simulink model "Modified"  (R2014b)
settings: Solver=ode23s  StartTime=0.0  StopTime=30  FixedStep=0.001  MaxStep=0.01  RelTol=1e-3
StopFcn:
  | plotting
values from neighbouring files (symbols this model uses):
  Par =     [init_params.mat]
undefined symbols (not defined in the file or in its folder): sigbuilder_block
libraries: simulink x4
(part 1 of 2)
settings Model: DSRTSU_INTERNAL_RTI_VER=440  DSRTSU_INTERNAL_RTI_TYPE=rti1401  RTICANMMDATA=struct('GeneralSetupData',struct('modelroot','D:\Users\bengtja\Subversion_work\TM_VEAS_VD\CourseMaterial\MMF062_VehicleDynamics\Compendium\AllPurposeModel','generalsettings',struct('filesettings',struct('destfolder',struct('Name','RTICANMM_FILES','Check',1),'buildfolder',struct('Name','.','Check',1),'AbsDestfolder',struct('Name','D:\Users\bengtja\Subversion_work\TM_VEAS_VD\CourseMaterial\MMF062_VehicleDynamics\Compendium\AllPurposeModel\RTICANMM_FILES'),'AbsBuildfolder',struct('Name','D:\Users\bengtja\Subversion_work\TM_VEAS_VD\CourseMaterial\MMF062_VehicleDynamics\Compendium\AllPurposeModel'))),'options',struct('addpaths',1,'rmpaths',1,'addtrcexclusion',logical(1),'cannavigator',struct('checkmonitoring',0),'show_usrtrc',0,'use_usrtrc',0),'advanced',struct('options',[1 1 1 1 1 1 1 1 1 1 1 1 1 1 1 1 1 1 1 1 1 1 1 1 1 1 1 1 1 1 1 1 1 1 1 1 1 1 1 1 1 1 1 1 1 1 1 1 1 1 1 1 1 1 1 1 1 1 1 1 1 1 1 1 1 1 1 1 1 1 1 1 1 1 1 1 1 1 1 1 1 1 1 1 1 1 1 1 1 1 1 1 1 1 1 1 1 1 1 1]),'MPSetup',{{}},'modelname','AllPurposeModel','block','AllPurposeModel'))  DSRTSU_INTERNAL_RTIFPGA=30  BufferReuse=off  Creator=bengtja  LastModifiedBy=danielpihlquist
settings OptimizationCC: BlockReduction=off  OptimizeBlockIOStorage=off  BufferReuse=off  GlobalBufferReuse=off  ExpressionFolding=off  LocalBlockOutputs=off
settings DebuggingCC: ArtificialAlgebraicLoopMsg=none  UnderspecifiedInitializationDetection=Classic  MergeDetectMultiDrivingBlocksExec=none  StateNameClashWarn=warning
settings HardwareCC: ProdIntDivRoundTo=Zero  ProdEndianess=BigEndian  ProdHWDeviceType=Generic->Custom  TargetIntDivRoundTo=Zero  TargetEndianess=BigEndian  TargetHWDeviceType=Generic->Custom
settings RTWCC: SystemTargetFile=rti1401.tlc  MakeCommand=make_rti  TemplateMakefile=rti1401.tmf  Description=dSPACE DS1401 Hardware Platform  ProcessScript=rti1401_make_rtw_hook
settings STFCustomTargetCC: ParMdlRefBuildCompliant=on  GeneratePreprocessorConditionals=Disable all  MatFileLogging=on  CPPClassGenCompliant=on  SystemTargetFile=rti1401.tlc
settings GRTTargetCC: CompOptLevelCompliant=off  ConcurrentExecutionCompliant=off  CombineOutputUpdateFcns=off  GRTInterface=on  ExtModeMexFile=noextcomm

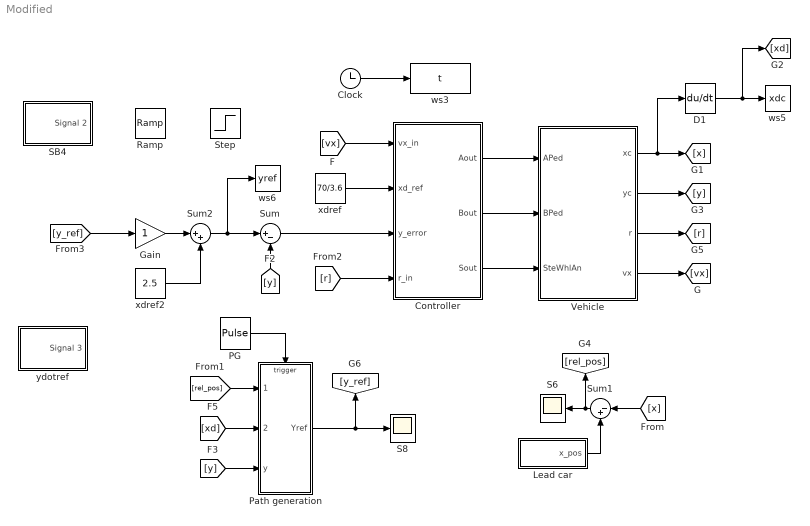
== system Modified ==
  Clock : Clock
  Controller : Subsystem
  D1 : Derivative
  Gain : Gain
  Lead car : Subsystem
  PG : DiscretePulseGenerator  PulseType=Time based  Period=1  PulseWidth=5
  Path generation : Subsystem
  Ramp : simulink/Sources/Ramp  slope=1  start=1  X0=0
  S6 : Scope
      settings: YMin=0  YMax=9  SaveName=ScopeData8
  S8 : Scope
      settings: YMin=0  YMax=9  SaveName=ScopeData10
  SB4 : Subsystem  Tag=STV Subsys  LoadFcn=sigbuilder_block('load');  StartFcn=sigbuilder_block('start');  StopFcn=sigbuilder_block('stop');  ClipboardFcn=sigbuilder_block('clipboard');  mask(Sigbuilder block){}
      mask help: Simulink:masks:SigbuilderBlock_MD
      mask init:
      | if ~strcmp(get_param(bdroot(gcbh),'SimulationStatus'),'stopped') tuvar = sigbuilder_block('maskInit'); end
      settings: CopyFcn=sigbuilder_block('copy');  DeleteFcn=sigbuilder_block('delete');  ModelCloseFcn=sigbuilder_block('modelClose');  PreSaveFcn=sigbuilder_block('preSave');  PauseFcn=sigbuilder_block('pause');  ContinueFcn=sigbuilder_block('continue');  NameChangeFcn=sigbuilder_block('namechange');  OpenFcn=sigbuilder_block('open',[437.6 199.2 550.4 400 ]);  CloseFcn=sigbuilder_block('close');
      mask Display: plot(0, 0, 100, 100,[2, 2, 32, 32, 2], [68, 8, 8, 68, 68],[32, 2], [38, 38], [32, 19, 2],[53, 60, 44], [32, 17, 17, 2],[16, 16, 31, 31]);txt = getActiveGroup(gcbh);text(2, 100, txt,'verticalAlignment', 'top');
  Step : Step  SampleTime=0
  Sum : Sum  Inputs=|+-
  Sum1 : Sum  Inputs=|-+
  Sum2 : Sum  Inputs=|++
  Vehicle : Subsystem
  ws3 : ToWorkspace  VariableName=t  SampleTime=-1
  ws5 : ToWorkspace  VariableName=xdc  SampleTime=-1
  ws6 : ToWorkspace  VariableName=yref  SampleTime=-1
  xdref : Constant  Value=70/3.6
  xdref2 : Constant  Value=2.5
  ydotref : Subsystem  Tag=STV Subsys  LoadFcn=sigbuilder_block('load');  StartFcn=sigbuilder_block('start');  StopFcn=sigbuilder_block('stop');  ClipboardFcn=sigbuilder_block('clipboard');  mask(Sigbuilder block){}
      mask help: Simulink:masks:SigbuilderBlock_MD
      mask init:
      | if ~strcmp(get_param(bdroot(gcbh),'SimulationStatus'),'stopped') tuvar = sigbuilder_block('maskInit'); end
      settings: CopyFcn=sigbuilder_block('copy');  DeleteFcn=sigbuilder_block('delete');  ModelCloseFcn=sigbuilder_block('modelClose');  PreSaveFcn=sigbuilder_block('preSave');  PauseFcn=sigbuilder_block('pause');  ContinueFcn=sigbuilder_block('continue');  NameChangeFcn=sigbuilder_block('namechange');  OpenFcn=sigbuilder_block('open',[437.6 199.2 550.4 400 ]);  CloseFcn=sigbuilder_block('close');
      mask Display: plot(0, 0, 100, 100,[2, 2, 32, 32, 2], [68, 8, 8, 68, 68],[32, 2], [38, 38], [32, 19, 2],[53, 60, 44], [32, 17, 17, 2],[16, 16, 31, 31]);txt = getActiveGroup(gcbh);text(2, 100, txt,'verticalAlignment', 'top');
  wires:
  Clock/1 -> ws3/1
  D1/1 -> ws5/1, [xd]
  Path generation/1(Yref) -> S8/1, [y_ref]
  Sum1/1 -> S6/1, [rel_pos]
  PG/1 -> Path generation/Trigger
  Gain/1 -> Sum2/1
  Sum2/1 -> ws6/1, Sum/1
  xdref2/1 -> Sum2/2
  Lead car/1(x_pos) -> Sum1/2
  xdref/1 -> Controller/2(xd_ref)
  Sum/1 -> Controller/3(y_error)
  [vx] -> Controller/1(vx_in)
  [y] -> Sum/2
  [y] -> Path generation/3(y)
  [xd] -> Path generation/2(xDot)
  [rel_pos] -> Path generation/1(RelPos)
  [r] -> Controller/4(r_in)
  [x] -> Sum1/1
  Vehicle/1(xc) -> D1/1, [x]
  Controller/1(Aout) -> Vehicle/1(APed)
  Controller/2(Bout) -> Vehicle/2(BPed)
  Controller/3(Sout) -> Vehicle/3(SteWhlAn)
  Vehicle/2(yc) -> [y]
  Vehicle/3(r) -> [r]
  Vehicle/4(vx) -> [vx]
  [y_ref] -> Gain/1

== system Modified/Controller ==
  vx_in : Inport
  xd_ref : Inport  Port=2
  y_error : Inport  Port=3
  r_in : Inport  Port=4
  Cartesian controller : Subsystem
  PID2 : simulink/Continuous/PID Controller  Controller=PID  TimeDomain=Continuous-time  SampleTime=-1  IntegratorMethod=Forward Euler  FilterMethod=Forward Euler  Form=Parallel  P=2  I=1  D=0.1  N=0  InitialConditionSource=internal  InitialConditionForIntegrator=0  InitialConditionForFilter=0  ExternalReset=none  LimitOutput=off  UpperSaturationLimit=inf  LowerSaturationLimit=-inf  LinearizeAsGain=on  AntiWindupMode=none  Kb=1  TrackingMode=off  Kt=1  PParamMin=[]  PParamMax=[]  IParamMin=[]  IParamMax=[]  DParamMin=[]  DParamMax=[]  NParamMin=[]  NParamMax=[]  KbParamMin=[]  KbParamMax=[]  KtParamMin=[]  KtParamMax=[]  POutMin=[]  POutMax=[]  IOutMin=[]  IOutMax=[]  DOutMin=[]  DOutMax=[]  NOutMin=[]  NOutMax=[]  KbOutMin=[]  KbOutMax=[]  KtOutMin=[]  KtOutMax=[]  IntegratorOutMin=[]  IntegratorOutMax=[]  FilterOutMin=[]  FilterOutMax=[]  SumOutMin=[]  SumOutMax=[]  SumI1OutMin=[]  SumI1OutMax=[]  SumI2OutMin=[]  SumI2OutMax=[]  SumI3OutMin=[]  SumI3OutMax=[]  SumDOutMin=[]  SumDOutMax=[]  SaturationOutMin=[]  SaturationOutMax=[]  IntegratorContinuousStateAttributes=''  IntegratorStateMustResolveToSignalObject=off  IntegratorRTWStateStorageClass=Auto  FilterContinuousStateAttributes=''  FilterStateMustResolveToSignalObject=off  FilterRTWStateStorageClass=Auto  DifferentiatorICPrevScaledInput=0  DifferentiatorOutMin=[]  DifferentiatorOutMax=[]  UseFilter=on
  Velocity and angle controller : Subsystem
  Aout : Outport
  Bout : Outport  Port=2
  Sout : Outport  Port=3
  wires:
  xd_ref/1 -> Cartesian controller/2(xcd_ref)
  Cartesian controller/2(r_ref) -> Velocity and angle controller/3(r_ref)
  Cartesian controller/1(vx_ref) -> Velocity and angle controller/2(vx_ref)
  r_in/1 -> Velocity and angle controller/4(r_in), Cartesian controller/3(r_in)
  Velocity and angle controller/1(Aout) -> Aout/1
  Velocity and angle controller/2(Bout) -> Bout/1
  Velocity and angle controller/3(Sout) -> Sout/1
  vx_in/1 -> Velocity and angle controller/1(vx_in), Cartesian controller/1(vx_in)
  PID2/1 -> Cartesian controller/4(ycd_ref)
  y_error/1 -> PID2/1

== system Modified/Lead car ==
  Integrator : Integrator  InitialCondition=50
  ws8 : ToWorkspace  VariableName=fcar  SampleTime=-1
  xdref1 : Constant  Value=60/3.6
  x_pos : Outport
  wires:
  xdref1/1 -> Integrator/1
  Integrator/1 -> x_pos/1, ws8/1

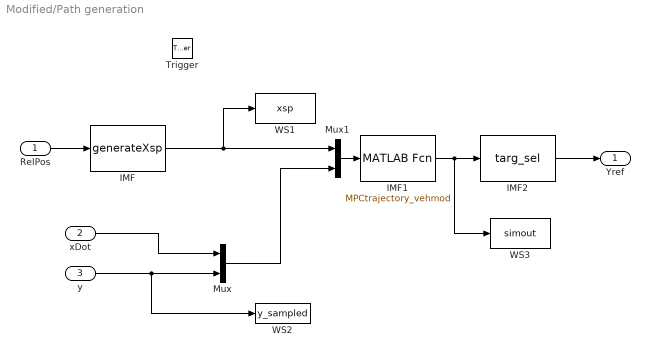
== system Modified/Path generation ==
  RelPos : Inport
  xDot : Inport  Port=2
  y : Inport  Port=3
  Trigger : TriggerPort  PortDimensions=1
  IMF : MATLABFcn  MATLABFcn=generateXsp
  IMF1 : MATLABFcn  MATLABFcn=MPCtrajectory_vehmod
  IMF2 : MATLABFcn  MATLABFcn=targ_sel
  Mux : Mux  Inputs=2
  Mux1 : Mux  Inputs=2
  WS1 : ToWorkspace  VariableName=xsp  SampleTime=-1
  WS2 : ToWorkspace  VariableName=y_sampled  SampleTime=-1
  WS3 : ToWorkspace  VariableName=simout  SampleTime=-1
  Yref : Outport
  wires:
  Mux1/1 -> IMF1/1
  Mux/1 -> Mux1/2
  IMF/1 -> WS1/1, Mux1/1
  RelPos/1 -> IMF/1
  xDot/1 -> Mux/1
  IMF2/1 -> Yref/1
  IMF1/1 -> IMF2/1, WS3/1
  y/1 -> WS2/1, Mux/2

== system Modified/SB4 ==
  Demux : Demux  Tag=STV Demux  Outputs=1
  FromWs : FromWorkspace  Tag=STV FromWs  VariableName=tuvar  SampleTime=0
      SigBuilderData=|
      | common.afterFinalStr = 'Extrapolate'
      | common.sampleTime = 0
      | dataSet.timeRange = [0 10]
      | dataSet.name = 'Group 1'
      | sbobj.Groups.Name = 'Group 1'
      | sbobj.Groups.Signals.Name = 'Signal 2'
      | sbobj.Groups.Signals.XData = [0 0.5 0.5 1 1 1.5 1.5 2 2 2.5 2.5 3 3 3.5 3.5 4 4 4.5 4.5 5 5 5.5 5.5 6 6 6.5 6.5 7 7 7.5 7.5 8 8 8.5 8.5 9 9.5 10]
      | sbobj.Groups.Signals.YData = [0 0 0.275 0.275 0.58 0.58 1 1 1.005 1.005 0.995 0.995 0.745 0.745 0.505 0.505 0.18 0.18 -0.305 -0.305 -0.425 -0.425 -0.56 -0.56 -0.52 -0.52 -0.46 -0.46 -0.43 -0.43 -0.28 -0.28 -0.21 -0.21 0 0 0 0]
  Signal 2 : Outport  Tag=STV Outport
  wires:
  Demux/1 -> Signal 2/1
  FromWs/1 -> Demux/1

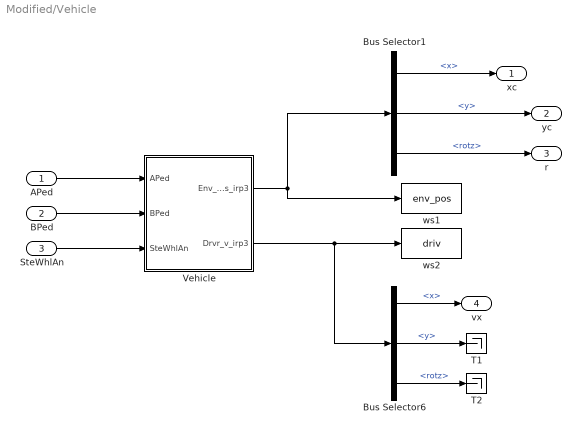
== system Modified/Vehicle ==
  APed : Inport
  BPed : Inport  Port=2
  SteWhlAn : Inport  Port=3
  Bus Selector1 : BusSelector  OutputSignals=x,y,rotz
  Bus Selector6 : BusSelector  OutputSignals=x,y,rotz
  T1 : Terminator
  T2 : Terminator
  Vehicle : Subsystem
  ws1 : ToWorkspace  VariableName=env_pos  SaveFormat=Timeseries  SampleTime=-1
  ws2 : ToWorkspace  VariableName=driv  SaveFormat=Timeseries  SampleTime=-1
  xc : Outport
  yc : Outport  Port=2
  r : Outport  Port=3
  vx : Outport  Port=4
  wires:
  Bus Selector1/1 -> xc/1  "<x>"
  Vehicle/1(Env_pos_irp3) -> Bus Selector1/1, ws1/1
  Vehicle/2(Drvr_v_irp3) -> ws2/1, Bus Selector6/1
  Bus Selector1/2 -> yc/1  "<y>"
  SteWhlAn/1 -> Vehicle/3(SteWhlAn)
  BPed/1 -> Vehicle/2(BPed)
  APed/1 -> Vehicle/1(APed)
  Bus Selector1/3 -> r/1  "<rotz>"
  Bus Selector6/1 -> vx/1  "<x>"
  Bus Selector6/2 -> T1/1  "<y>"
  Bus Selector6/3 -> T2/1  "<rotz>"

== system Modified/ydotref ==
  Demux : Demux  Tag=STV Demux  Outputs=1
  FromWs : FromWorkspace  Tag=STV FromWs  VariableName=tuvar  SampleTime=0
      SigBuilderData=|
      | common.afterFinalStr = 'Extrapolate'
      | common.sampleTime = 0
      | dataSet.timeRange = [0 10]
      | dataSet.name = 'Group 1'
      | sbobj.Groups.Name = 'Group 1'
      | sbobj.Groups.Signals.Name = 'Signal 3'
      | sbobj.Groups.Signals.XData = [0 0.5 0.5 6.8 7.9 8.3 9.26 10]
      | sbobj.Groups.Signals.YData = [0 0 1 1 1 1 1 1]
  Signal 3 : Outport  Tag=STV Outport
  wires:
  Demux/1 -> Signal 3/1
  FromWs/1 -> Demux/1

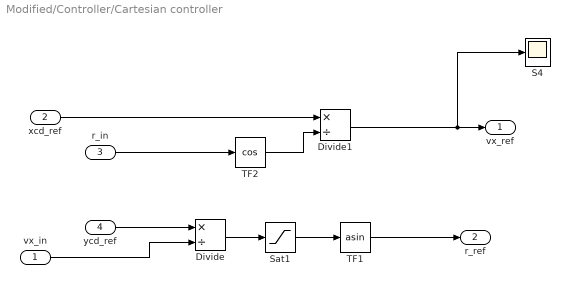
== system Modified/Controller/Cartesian controller ==
  vx_in : Inport
  xcd_ref : Inport  Port=2
  r_in : Inport  Port=3
  ycd_ref : Inport  Port=4
  Divide : Product  Inputs=*/
  Divide1 : Product  Inputs=*/
  S4 : Scope
      settings: SaveName=ScopeData4
  Sat1 : Saturate  UpperLimit=1  LowerLimit=-1
  TF1 : Trigonometry  Operator=asin
  TF2 : Trigonometry  Operator=cos
  vx_ref : Outport
  r_ref : Outport  Port=2
  wires:
  xcd_ref/1 -> Divide1/1
  TF2/1 -> Divide1/2
  r_in/1 -> TF2/1
  vx_in/1 -> Divide/2
  Divide/1 -> Sat1/1
  TF1/1 -> r_ref/1
  Sat1/1 -> TF1/1
  ycd_ref/1 -> Divide/1
  Divide1/1 -> S4/1, vx_ref/1

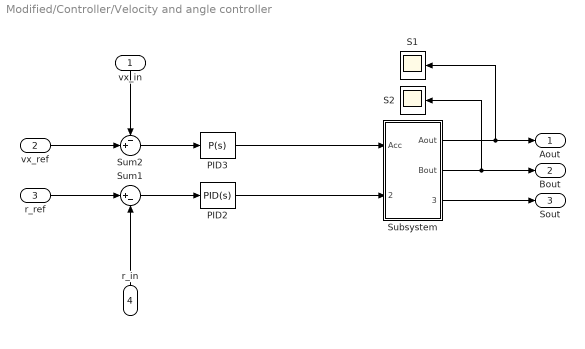
== system Modified/Controller/Velocity and angle controller ==
  vx_in : Inport
  vx_ref : Inport  Port=2
  r_ref : Inport  Port=3
  r_in : Inport  Port=4
  PID2 : simulink/Continuous/PID Controller  Controller=PID  TimeDomain=Continuous-time  SampleTime=-1  IntegratorMethod=Forward Euler  FilterMethod=Forward Euler  Form=Parallel  P=5000  I=1  D=0  N=100  InitialConditionSource=internal  InitialConditionForIntegrator=0  InitialConditionForFilter=0  ExternalReset=none  LimitOutput=off  UpperSaturationLimit=inf  LowerSaturationLimit=-inf  LinearizeAsGain=on  AntiWindupMode=none  Kb=1  TrackingMode=off  Kt=1  PParamMin=[]  PParamMax=[]  IParamMin=[]  IParamMax=[]  DParamMin=[]  DParamMax=[]  NParamMin=[]  NParamMax=[]  KbParamMin=[]  KbParamMax=[]  KtParamMin=[]  KtParamMax=[]  POutMin=[]  POutMax=[]  IOutMin=[]  IOutMax=[]  DOutMin=[]  DOutMax=[]  NOutMin=[]  NOutMax=[]  KbOutMin=[]  KbOutMax=[]  KtOutMin=[]  KtOutMax=[]  IntegratorOutMin=[]  IntegratorOutMax=[]  FilterOutMin=[]  FilterOutMax=[]  SumOutMin=[]  SumOutMax=[]  SumI1OutMin=[]  SumI1OutMax=[]  SumI2OutMin=[]  SumI2OutMax=[]  SumI3OutMin=[]  SumI3OutMax=[]  SumDOutMin=[]  SumDOutMax=[]  SaturationOutMin=[]  SaturationOutMax=[]  IntegratorContinuousStateAttributes=''  IntegratorStateMustResolveToSignalObject=off  IntegratorRTWStateStorageClass=Auto  FilterContinuousStateAttributes=''  FilterStateMustResolveToSignalObject=off  FilterRTWStateStorageClass=Auto  DifferentiatorICPrevScaledInput=0  DifferentiatorOutMin=[]  DifferentiatorOutMax=[]  UseFilter=on
  PID3 : simulink/Continuous/PID Controller  Controller=P  TimeDomain=Continuous-time  SampleTime=-1  IntegratorMethod=Forward Euler  FilterMethod=Forward Euler  Form=Parallel  P=100  I=0  D=0  N=100  InitialConditionSource=internal  InitialConditionForIntegrator=0  InitialConditionForFilter=0  ExternalReset=none  LimitOutput=off  UpperSaturationLimit=inf  LowerSaturationLimit=-inf  LinearizeAsGain=on  AntiWindupMode=none  Kb=1  TrackingMode=off  Kt=1  PParamMin=[]  PParamMax=[]  IParamMin=[]  IParamMax=[]  DParamMin=[]  DParamMax=[]  NParamMin=[]  NParamMax=[]  KbParamMin=[]  KbParamMax=[]  KtParamMin=[]  KtParamMax=[]  POutMin=[]  POutMax=[]  IOutMin=[]  IOutMax=[]  DOutMin=[]  DOutMax=[]  NOutMin=[]  NOutMax=[]  KbOutMin=[]  KbOutMax=[]  KtOutMin=[]  KtOutMax=[]  IntegratorOutMin=[]  IntegratorOutMax=[]  FilterOutMin=[]  FilterOutMax=[]  SumOutMin=[]  SumOutMax=[]  SumI1OutMin=[]  SumI1OutMax=[]  SumI2OutMin=[]  SumI2OutMax=[]  SumI3OutMin=[]  SumI3OutMax=[]  SumDOutMin=[]  SumDOutMax=[]  SaturationOutMin=[]  SaturationOutMax=[]  IntegratorContinuousStateAttributes=''  IntegratorStateMustResolveToSignalObject=off  IntegratorRTWStateStorageClass=Auto  FilterContinuousStateAttributes=''  FilterStateMustResolveToSignalObject=off  FilterRTWStateStorageClass=Auto  DifferentiatorICPrevScaledInput=0  DifferentiatorOutMin=[]  DifferentiatorOutMax=[]  UseFilter=on
  S1 : Scope
      settings: YMin=0  YMax=9  SaveName=ScopeData6
  S2 : Scope
      settings: YMin=0  YMax=9  SaveName=ScopeData7
  Subsystem : Subsystem
  Sum1 : Sum  Inputs=|+-
  Sum2 : Sum  Inputs=-+|
  Aout : Outport
  Bout : Outport  Port=2
  Sout : Outport  Port=3
  wires:
  r_in/1 -> Sum1/2
  Sum1/1 -> PID2/1
  r_ref/1 -> Sum1/1
  Sum2/1 -> PID3/1
  vx_ref/1 -> Sum2/2
  vx_in/1 -> Sum2/1
  Subsystem/2(Bout) -> S2/1, Bout/1
  PID2/1 -> Subsystem/2(Steer)
  Subsystem/3(SOut) -> Sout/1
  PID3/1 -> Subsystem/1(Acc)
  Subsystem/1(Aout) -> S1/1, Aout/1

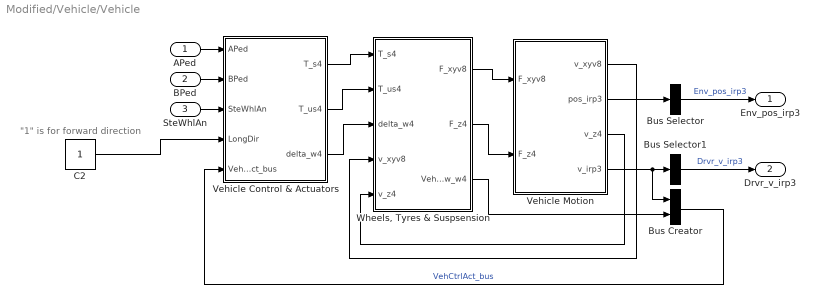
== system Modified/Vehicle/Vehicle ==
  note: "1" is for forward direction
  APed : Inport
  BPed : Inport  Port=2
  SteWhlAn : Inport  Port=3
  Bus Creator : BusCreator  Inputs=2
  Bus Selector : BusSelector  OutputSignals=x,y,rotz  OutputAsBus=on
  Bus Selector1 : BusSelector  OutputSignals=x,y,rotz  OutputAsBus=on
  C2 : Constant
  Vehicle Control & Actuators : Subsystem
  Vehicle Motion : Subsystem
  "Wheels, Tyres & Suspsension" : Subsystem
  Env_pos_irp3 : Outport
  Drvr_v_irp3 : Outport  Port=2
  wires:
  Vehicle Motion/2(pos_irp3) -> Bus Selector/1
  BPed/1 -> Vehicle Control & Actuators/2(BPed)
  SteWhlAn/1 -> Vehicle Control & Actuators/3(SteWhlAn)
  APed/1 -> Vehicle Control & Actuators/1(APed)
  Vehicle Control & Actuators/2(T_us4) -> "Wheels, Tyres & Suspsension"/2(T_us4)
  Vehicle Control & Actuators/1(T_s4) -> "Wheels, Tyres & Suspsension"/1(T_s4)
  Vehicle Control & Actuators/3(delta_w4) -> "Wheels, Tyres & Suspsension"/3(delta_w4)
  "Wheels, Tyres & Suspsension"/1(F_xyv8) -> Vehicle Motion/1(F_xyv8)
  "Wheels, Tyres & Suspsension"/2(F_z4) -> Vehicle Motion/2(F_z4)
  Vehicle Motion/1(v_xyv8) -> "Wheels, Tyres & Suspsension"/4(v_xyv8)
  Vehicle Motion/3(v_z4) -> "Wheels, Tyres & Suspsension"/5(v_z4)
  Vehicle Motion/4(v_irp3) -> Bus Creator/1, Bus Selector1/1
  "Wheels, Tyres & Suspsension"/3(VehCtrlAct_w_w4) -> Bus Creator/2
  Bus Creator/1 -> Vehicle Control & Actuators/5(VehCtrlAct_bus)  "VehCtrlAct_bus"
  Bus Selector/1 -> Env_pos_irp3/1  "Env_pos_irp3"
  Bus Selector1/1 -> Drvr_v_irp3/1  "Drvr_v_irp3"
  C2/1 -> Vehicle Control & Actuators/4(LongDir)

== system Modified/Controller/Velocity and angle controller/Subsystem ==
  Acc : Inport
  Steer : Inport  Port=2
  Gain : Gain  Gain=2/300
  Sat1 : Saturate  UpperLimit=10  LowerLimit=-10
  Sat2 : Saturate  UpperLimit=0  LowerLimit=-1
  Sat3 : Saturate  UpperLimit=1  LowerLimit=0
  Aout : Outport
  Bout : Outport  Port=2
  SOut : Outport  Port=3
  wires:
  Sat1/1 -> SOut/1
  Gain/1 -> Sat1/1
  Steer/1 -> Gain/1
  Acc/1 -> Sat3/1, Sat2/1
  Sat3/1 -> Aout/1
  Sat2/1 -> Bout/1

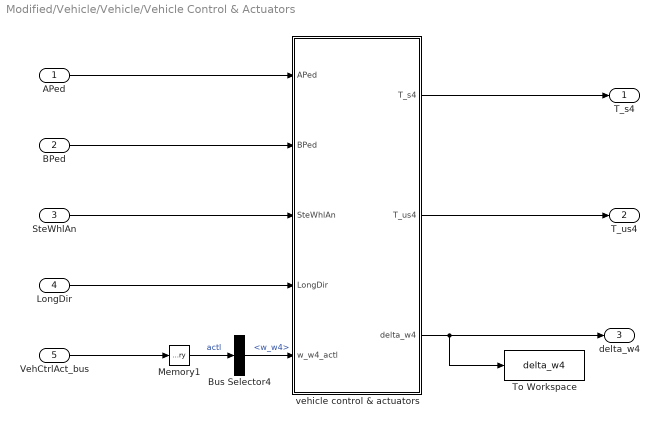
== system Modified/Vehicle/Vehicle/Vehicle Control & Actuators ==
  APed : Inport
  BPed : Inport  Port=2
  SteWhlAn : Inport  Port=3
  LongDir : Inport  Port=4
  VehCtrlAct_bus : Inport  Port=5
  Bus Selector4 : BusSelector  OutputSignals=VehCtrlAct_w_w4.w_w4
  Memory1 : Memory  X0=Par.Init.v_x
  To Workspace : ToWorkspace  VariableName=delta_w4  SaveFormat=Timeseries  SampleTime=-1
  vehicle control & actuators : MATLAB Function  TreatAsAtomicUnit=on
      settings: MinAlgLoopOccurrences=on
  T_s4 : Outport
  T_us4 : Outport  Port=2
  delta_w4 : Outport  Port=3
  wires:
  APed/1 -> vehicle control & actuators/1(APed)
  vehicle control & actuators/2(T_us4) -> T_us4/1
  BPed/1 -> vehicle control & actuators/2(BPed)
  SteWhlAn/1 -> vehicle control & actuators/3(SteWhlAn)
  vehicle control & actuators/1(T_s4) -> T_s4/1
  vehicle control & actuators/3(delta_w4) -> To Workspace/1, delta_w4/1
  VehCtrlAct_bus/1 -> Memory1/1
  Bus Selector4/1 -> vehicle control & actuators/5(w_w4_actl)  "<w_w4>"
  LongDir/1 -> vehicle control & actuators/4(LongDir)
  Memory1/1 -> Bus Selector4/1  "actl"

== system Modified/Vehicle/Vehicle/Vehicle Motion ==
  note: "Sprung Body OORP" could also output pos_oorp3 by integrating v_oorp3.
  F_xyv8 : Inport
  F_z4 : Inport  Port=2
  Compatibility IRP : Subsystem
  Compatibility OORP : Subsystem
  Sprung Body OORP : Subsystem
  Whole Vehicle IRP : Subsystem
  v_xyv8 : Outport
  pos_irp3 : Outport  Port=2
  v_z4 : Outport  Port=3
  v_irp3 : Outport  Port=4
  wires:
  F_xyv8/1 -> Whole Vehicle IRP/1(F_xyv8), Sprung Body OORP/1(F_xyv8)
  F_z4/1 -> Sprung Body OORP/2(F_z4)
  Sprung Body OORP/1(v_oorp3) -> Compatibility OORP/1(v_oorp3)
  Compatibility OORP/1(v_z4) -> v_z4/1
  Compatibility IRP/1(v_xyv8) -> v_xyv8/1
  Whole Vehicle IRP/1(v_irp3) -> v_irp3/1, Compatibility IRP/1(v_irp3)
  Whole Vehicle IRP/2(pos_irp3) -> pos_irp3/1

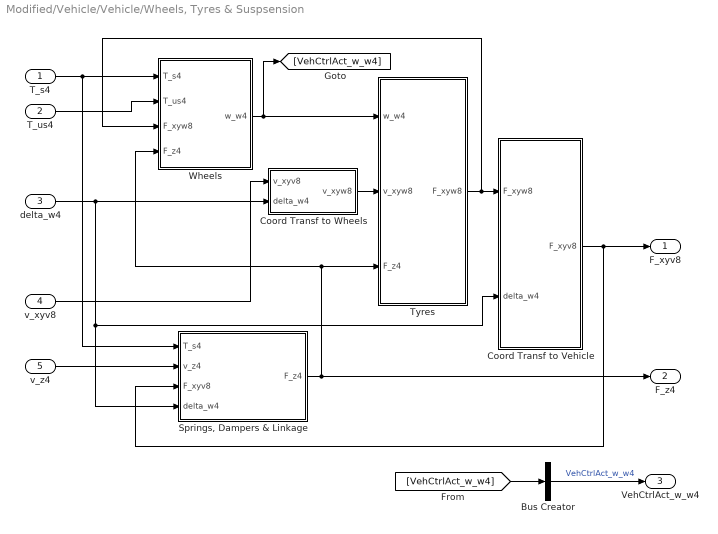
== system Modified/Vehicle/Vehicle/Wheels, Tyres & Suspsension ==
  T_s4 : Inport
  T_us4 : Inport  Port=2
  delta_w4 : Inport  Port=3
  v_xyv8 : Inport  Port=4
  v_z4 : Inport  Port=5
  Bus Creator : BusCreator  Inputs=1
  Coord Transf to Vehicle : Subsystem
      settings: MinAlgLoopOccurrences=on
  "Coord Transf to Wheels " : Subsystem
      settings: MinAlgLoopOccurrences=on
  "Springs, Dampers & Linkage" : Subsystem
      settings: MinAlgLoopOccurrences=on
  "Tyres " : Subsystem
      settings: MinAlgLoopOccurrences=on
  "Wheels " : Subsystem
      settings: MinAlgLoopOccurrences=on
  F_xyv8 : Outport
  F_z4 : Outport  Port=2
  VehCtrlAct_w_w4 : Outport  Port=3
  wires:
  "Tyres "/1(F_xyw8) -> "Wheels "/3(F_xyw8), Coord Transf to Vehicle/1(F_xyw8)
  "Coord Transf to Wheels "/1(v_xyw8) -> "Tyres "/2(v_xyw8)
  delta_w4/1 -> "Springs, Dampers & Linkage"/4(delta_w4), Coord Transf to Vehicle/2(delta_w4), "Coord Transf to Wheels "/2(delta_w4)
  "Wheels "/1(w_w4) -> [VehCtrlAct_w_w4], "Tyres "/1(w_w4)
  T_us4/1 -> "Wheels "/2(T_us4)
  v_xyv8/1 -> "Coord Transf to Wheels "/1(v_xyv8)
  Bus Creator/1 -> VehCtrlAct_w_w4/1  "VehCtrlAct_w_w4"
  [VehCtrlAct_w_w4] -> Bus Creator/1
  v_z4/1 -> "Springs, Dampers & Linkage"/2(v_z4)
  T_s4/1 -> "Springs, Dampers & Linkage"/1(T_s4), "Wheels "/1(T_s4)
  Coord Transf to Vehicle/1(F_xyv8) -> F_xyv8/1, "Springs, Dampers & Linkage"/3(F_xyv8)
  "Springs, Dampers & Linkage"/1(F_z4) -> F_z4/1, "Tyres "/3(F_z4), "Wheels "/4(F_z4)

== system Modified/Vehicle/Vehicle/Vehicle Motion/Compatibility IRP ==
  v_irp3 : Inport
  Bus Creator3 : BusCreator  Inputs=2
  Compatibility : MATLAB Function  TreatAsAtomicUnit=on
  To Workspace1 : ToWorkspace  VariableName=v_xv4  SaveFormat=Timeseries  SampleTime=-1
  To Workspace2 : ToWorkspace  VariableName=v_yv4  SaveFormat=Timeseries  SampleTime=-1
  v_xyv8 : Outport
  wires:
  v_irp3/1 -> Compatibility/1(v_irp3)
  Compatibility/1(v_xv4) -> Bus Creator3/1, To Workspace1/1
  Compatibility/2(v_yv4) -> Bus Creator3/2, To Workspace2/1
  Bus Creator3/1 -> v_xyv8/1  "v_xyv8"

== system Modified/Vehicle/Vehicle/Vehicle Motion/Compatibility OORP ==
  v_oorp3 : Inport
  Compatibility Eq [1.11] : MATLAB Function  TreatAsAtomicUnit=on
  v_z4 : Outport
  wires:
  v_oorp3/1 -> Compatibility Eq [1.11]/1(v_oorp3)
  Compatibility Eq [1.11]/1(v_z4) -> v_z4/1

== system Modified/Vehicle/Vehicle/Vehicle Motion/Sprung Body OORP ==
  F_xyv8 : Inport
  F_z4 : Inport  Port=2
  Body OORP : MATLAB Function  TreatAsAtomicUnit=on
  Bus Selector1 : BusSelector  OutputSignals=F_xv4,F_yv4
  Integrator : Subsystem
  v_oorp3 : Outport
  wires:
  F_z4/1 -> Body OORP/3(F_z4)
  Body OORP/1(derv_oorp3) -> Integrator/1(derv_z)
  Integrator/1(v_oorp3) -> v_oorp3/1
  F_xyv8/1 -> Bus Selector1/1
  Bus Selector1/1 -> Body OORP/1(F_xv4)  "<F_xv4>"
  Bus Selector1/2 -> Body OORP/2(F_yv4)  "<F_yv4>"

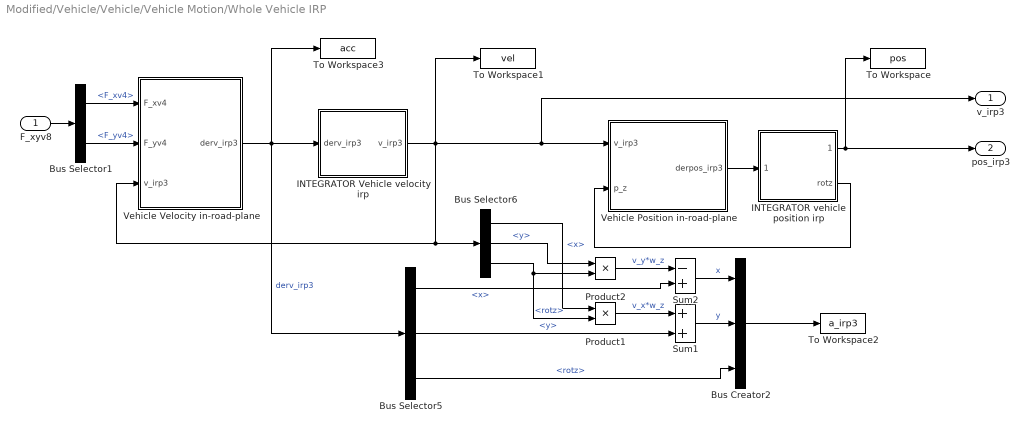
== system Modified/Vehicle/Vehicle/Vehicle Motion/Whole Vehicle IRP ==
  F_xyv8 : Inport
  Bus Creator2 : BusCreator  Inputs=3  OutDataTypeStr=Bus: irp_vec3
  Bus Selector1 : BusSelector  OutputSignals=F_xv4,F_yv4
  Bus Selector5 : BusSelector  OutputSignals=x,y,rotz
  Bus Selector6 : BusSelector  OutputSignals=x,y,rotz
  INTEGRATOR Vehicle velocity irp : Subsystem
  INTEGRATOR vehicle position irp : Subsystem
  Product1 : Product
  Product2 : Product
  Sum1 : Sum
  Sum2 : Sum  Inputs=-+
  To Workspace : ToWorkspace  VariableName=pos  SaveFormat=Timeseries  SampleTime=-1
  To Workspace1 : ToWorkspace  VariableName=vel  SaveFormat=Timeseries  SampleTime=-1
  To Workspace2 : ToWorkspace  VariableName=a_irp3  SaveFormat=Timeseries  SampleTime=-1
  To Workspace3 : ToWorkspace  VariableName=acc  SaveFormat=Timeseries  SampleTime=-1
  Vehicle Position in-road-plane : MATLAB Function  TreatAsAtomicUnit=on
  Vehicle Velocity in-road-plane : MATLAB Function  TreatAsAtomicUnit=on
  v_irp3 : Outport
  pos_irp3 : Outport  Port=2
  wires:
  Bus Creator2/1 -> To Workspace2/1
  Product1/1 -> Sum1/1  "v_x*w_z"
  Sum1/1 -> Bus Creator2/2  "y"
  Sum2/1 -> Bus Creator2/1  "x"
  Product2/1 -> Sum2/1  "v_y*w_z"
  Vehicle Velocity in-road-plane/1(derv_irp3) -> To Workspace3/1, Bus Selector5/1, INTEGRATOR Vehicle velocity irp/1(derv_irp3)  "derv_irp3"
  INTEGRATOR Vehicle velocity irp/1(v_irp3) -> Vehicle Position in-road-plane/1(v_irp3), v_irp3/1, Bus Selector6/1, Vehicle Velocity in-road-plane/3(v_irp3), To Workspace1/1
  Bus Selector5/3 -> Bus Creator2/3  "<rotz>"
  Bus Selector5/2 -> Sum1/2  "<y>"
  Bus Selector5/1 -> Sum2/2  "<x>"
  Bus Selector6/2 -> Product2/1  "<y>"
  Bus Selector6/3 -> Product2/2, Product1/2  "<rotz>"
  Bus Selector6/1 -> Product1/1  "<x>"
  INTEGRATOR vehicle position irp/1(pos_irp3) -> To Workspace/1, pos_irp3/1
  Vehicle Position in-road-plane/1(derpos_irp3) -> INTEGRATOR vehicle position irp/1(derpos_irp3)
  INTEGRATOR vehicle position irp/2(rotz) -> Vehicle Position in-road-plane/2(p_z)
  F_xyv8/1 -> Bus Selector1/1
  Bus Selector1/1 -> Vehicle Velocity in-road-plane/1(F_xv4)  "<F_xv4>"
  Bus Selector1/2 -> Vehicle Velocity in-road-plane/2(F_yv4)  "<F_yv4>"

== system Modified/Vehicle/Vehicle/Wheels, Tyres & Suspsension/Coord Transf to Vehicle ==
  F_xyw8 : Inport
  delta_w4 : Inport  Port=2
  Bus Creator3 : BusCreator  Inputs=2
  Bus Selector1 : BusSelector  OutputSignals=F_xw4,F_yw4
  Coord Transf to veh : MATLAB Function  TreatAsAtomicUnit=on
      settings: MinAlgLoopOccurrences=on
  F_xyv8 : Outport
  wires:
  delta_w4/1 -> Coord Transf to veh/3(delta_w4)
  Coord Transf to veh/1(F_xv4) -> Bus Creator3/1
  Coord Transf to veh/2(F_yv4) -> Bus Creator3/2
  F_xyw8/1 -> Bus Selector1/1
  Bus Creator3/1 -> F_xyv8/1  "F_xyv8"
  Bus Selector1/1 -> Coord Transf to veh/1(F_xw4)  "<F_xw4>"
  Bus Selector1/2 -> Coord Transf to veh/2(F_yw4)  "<F_yw4>"

== system Modified/Vehicle/Vehicle/Wheels, Tyres & Suspsension/Coord Transf to Wheels  ==
  v_xyv8 : Inport
  delta_w4 : Inport  Port=2
  Bus Creator4 : BusCreator  Inputs=2
  Bus Selector : BusSelector  OutputSignals=v_xv4,v_yv4
  Coord Transf to whl : MATLAB Function  TreatAsAtomicUnit=on
  v_xyw8 : Outport
  wires:
  v_xyv8/1 -> Bus Selector/1
  delta_w4/1 -> Coord Transf to whl/3(delta_w4)
  Bus Selector/1 -> Coord Transf to whl/1(v_xv4)  "<v_xv4>"
  Bus Selector/2 -> Coord Transf to whl/2(v_yv4)  "<v_yv4>"
  Bus Creator4/1 -> v_xyw8/1
  Coord Transf to whl/2(v_yw4) -> Bus Creator4/2
  Coord Transf to whl/1(v_xw4) -> Bus Creator4/1

== system Modified/Vehicle/Vehicle/Wheels, Tyres & Suspsension/Springs, Dampers & Linkage ==
  T_s4 : Inport
  v_z4 : Inport  Port=2
  F_xyv8 : Inport  Port=3
  delta_w4 : Inport  Port=4
  Bus Selector1 : BusSelector  OutputSignals=F_xv4,F_yv4
  Dampers : MATLAB Function  TreatAsAtomicUnit=on
      settings: MinAlgLoopOccurrences=on
  INTEGRATOR : Subsystem
  Springs : MATLAB Function  TreatAsAtomicUnit=on
      settings: MinAlgLoopOccurrences=on
  Sum : Subsystem
      settings: MinAlgLoopOccurrences=on
  Suspension Equilibrium : MATLAB Function  TreatAsAtomicUnit=on
      settings: MinAlgLoopOccurrences=on
  F_z4 : Outport
  wires:
  T_s4/1 -> Suspension Equilibrium/1(T_s4)
  v_z4/1 -> Dampers/1(v_z4), Springs/1(v_z4)
  Springs/1(derF_s4) -> INTEGRATOR/1(derF_s4)
  INTEGRATOR/1(F_4) -> Sum/1(F_s4)
  Sum/1(F_sd4) -> Suspension Equilibrium/2(F_sd4)
  Suspension Equilibrium/1(F_z4) -> F_z4/1
  Bus Selector1/1 -> Suspension Equilibrium/3(F_xv4)  "<F_xv4>"
  Bus Selector1/2 -> Suspension Equilibrium/4(F_yv4)  "<F_yv4>"
  Dampers/1(F_d4) -> Sum/2(F_d4)
  F_xyv8/1 -> Bus Selector1/1
  delta_w4/1 -> Suspension Equilibrium/5(delta_w4)

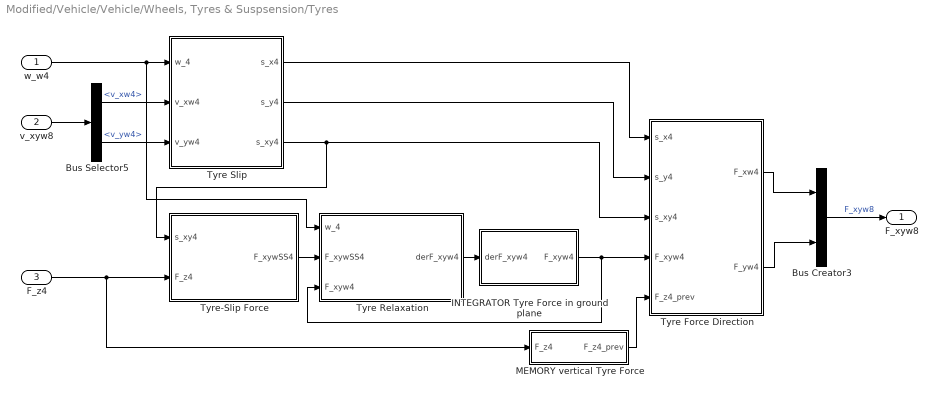
== system Modified/Vehicle/Vehicle/Wheels, Tyres & Suspsension/Tyres  ==
  w_w4 : Inport
  v_xyw8 : Inport  Port=2
  F_z4 : Inport  Port=3
  " MEMORY vertical Tyre Force" : Subsystem
      settings: MinAlgLoopOccurrences=on
  Bus Creator3 : BusCreator  Inputs=2
  Bus Selector5 : BusSelector  OutputSignals=v_xw4,v_yw4
  INTEGRATOR Tyre Force in ground plane : Subsystem
      settings: MinAlgLoopOccurrences=on
  Tyre Force Direction : MATLAB Function
  Tyre Relaxation : MATLAB Function  TreatAsAtomicUnit=on
      settings: MinAlgLoopOccurrences=on
  Tyre Slip : MATLAB Function  TreatAsAtomicUnit=on
      settings: MinAlgLoopOccurrences=on
  Tyre-Slip Force : MATLAB Function  TreatAsAtomicUnit=on
      settings: MinAlgLoopOccurrences=on
  F_xyw8 : Outport
  wires:
  w_w4/1 -> Tyre Relaxation/1(w_4), Tyre Slip/1(w_4)
  v_xyw8/1 -> Bus Selector5/1
  Tyre Slip/1(s_x4) -> Tyre Force Direction/1(s_x4)
  Tyre Slip/2(s_y4) -> Tyre Force Direction/2(s_y4)
  Bus Creator3/1 -> F_xyw8/1  "F_xyw8"
  Tyre Relaxation/1(derF_xyw4) -> INTEGRATOR Tyre Force in ground plane/1(derF_xyw4)
  INTEGRATOR Tyre Force in ground plane/1(F_xyw4) -> Tyre Force Direction/4(F_xyw4), Tyre Relaxation/3(F_xyw4)
  Tyre Force Direction/1(F_xw4) -> Bus Creator3/1
  Tyre Force Direction/2(F_yw4) -> Bus Creator3/2
  Tyre Slip/3(s_xy4) -> Tyre Force Direction/3(s_xy4), Tyre-Slip Force/1(s_xy4)
  Bus Selector5/1 -> Tyre Slip/2(v_xw4)  "<v_xw4>"
  Bus Selector5/2 -> Tyre Slip/3(v_yw4)  "<v_yw4>"
  Tyre-Slip Force/1(F_xywSS4) -> Tyre Relaxation/2(F_xywSS4)
  F_z4/1 -> " MEMORY vertical Tyre Force"/1(F_z4), Tyre-Slip Force/2(F_z4)
  " MEMORY vertical Tyre Force"/1(F_z4_prev) -> Tyre Force Direction/5(F_z4_prev)

== system Modified/Vehicle/Vehicle/Wheels, Tyres & Suspsension/Wheels  ==
  T_s4 : Inport
  T_us4 : Inport  Port=2
  F_xyw8 : Inport  Port=3
  F_z4 : Inport  Port=4
  Bus Selector1 : BusSelector  OutputSignals=F_xw4,F_yw4
  INTEGRATOR : Subsystem
  "Wheels " : MATLAB Function  TreatAsAtomicUnit=on
  w_w4 : Outport
  wires:
  T_us4/1 -> "Wheels "/2(T_us4)
  T_s4/1 -> "Wheels "/1(T_s4)
  "Wheels "/1(derw_w4) -> INTEGRATOR/1(derw_w4)
  F_z4/1 -> "Wheels "/5(F_z4)
  F_xyw8/1 -> Bus Selector1/1
  Bus Selector1/2 -> "Wheels "/4(F_yv4)  "<F_yw4>"
  Bus Selector1/1 -> "Wheels "/3(F_xv4)  "<F_xw4>"
  INTEGRATOR/1(w_w4) -> w_w4/1, "Wheels "/6(w_w4)

== system Modified/Vehicle/Vehicle/Vehicle Motion/Sprung Body OORP/Integrator ==
  derv_z : Inport
  Bus Creator : BusCreator  Inputs=3  OutDataTypeStr=Bus: oorp_vec3
  Bus Selector4 : BusSelector  OutputSignals=z,rotx,roty
  Integ Heave : Integrator
  Integ Pitch : Integrator
  Integ Roll : Integrator
  v_oorp3 : Outport
  wires:
  Integ Pitch/1 -> Bus Creator/3  "roty"
  Integ Heave/1 -> Bus Creator/1  "z"
  Integ Roll/1 -> Bus Creator/2  "rotx"
  Bus Creator/1 -> v_oorp3/1  "v_oorp3"
  derv_z/1 -> Bus Selector4/1
  Bus Selector4/1 -> Integ Heave/1  "<z>"
  Bus Selector4/2 -> Integ Roll/1  "<rotx>"
  Bus Selector4/3 -> Integ Pitch/1  "<roty>"

== system Modified/Vehicle/Vehicle/Vehicle Motion/Whole Vehicle IRP/INTEGRATOR Vehicle velocity irp ==
  derv_irp3 : Inport
  Bus Creator : BusCreator  Inputs=3  OutDataTypeStr=Bus: irp_vec3
  Bus Selector : BusSelector  OutputSignals=x,y,rotz
  Integ Lat : Integrator
  Integ Long : Integrator  InitialCondition=Par.Init.v_x
  Integ Yaw : Integrator
  v_irp3 : Outport
  wires:
  Bus Creator/1 -> v_irp3/1  "v_irp3"
  Bus Selector/3 -> Integ Yaw/1  "<rotz>"
  Bus Selector/1 -> Integ Long/1  "<x>"
  Integ Long/1 -> Bus Creator/1  "x"
  derv_irp3/1 -> Bus Selector/1
  Bus Selector/2 -> Integ Lat/1  "<y>"
  Integ Lat/1 -> Bus Creator/2  "y"
  Integ Yaw/1 -> Bus Creator/3  "rotz"

== system Modified/Vehicle/Vehicle/Vehicle Motion/Whole Vehicle IRP/INTEGRATOR vehicle position irp ==
  derpos_irp3 : Inport
  Bus Creator3 : BusCreator  Inputs=3  OutDataTypeStr=Bus: irp_vec3
  Bus Selector2 : BusSelector  OutputSignals=x,y,rotz
  Integ p_z : Integrator
  Integ x : Integrator
  Integ y : Integrator  InitialCondition=2.5
  pos_irp3 : Outport
  rotz : Outport  Port=2
  wires:
  derpos_irp3/1 -> Bus Selector2/1
  Integ y/1 -> Bus Creator3/2  "y"
  Integ p_z/1 -> rotz/1, Bus Creator3/3  "rotz"
  Integ x/1 -> Bus Creator3/1  "x"
  Bus Creator3/1 -> pos_irp3/1  "pos_irp3"
  Bus Selector2/3 -> Integ p_z/1  "<rotz>"
  Bus Selector2/1 -> Integ x/1  "<x>"
  Bus Selector2/2 -> Integ y/1  "<y>"

== system Modified/Vehicle/Vehicle/Wheels, Tyres & Suspsension/Springs, Dampers & Linkage/INTEGRATOR ==
  derF_s4 : Inport
  Bus Creator3 : BusCreator
  Bus Selector7 : BusSelector  OutputSignals=fl,fr,rl,rr
  Integrator1 : Integrator  InitialCondition=Par.Init.F_fz/2
  Integrator2 : Integrator  InitialCondition=Par.Init.F_fz/2
  Integrator3 : Integrator  InitialCondition=Par.Init.F_rz/2
  Integrator4 : Integrator  InitialCondition=Par.Init.F_rz/2
  F_4 : Outport
  wires:
  Integrator1/1 -> Bus Creator3/1  "fl"
  Integrator3/1 -> Bus Creator3/3  "rl"
  Integrator4/1 -> Bus Creator3/4  "rr"
  Integrator2/1 -> Bus Creator3/2  "fr"
  derF_s4/1 -> Bus Selector7/1
  Bus Selector7/1 -> Integrator1/1  "<fl>"
  Bus Creator3/1 -> F_4/1  "F_s4"
  Bus Selector7/2 -> Integrator2/1  "<fr>"
  Bus Selector7/4 -> Integrator4/1  "<rr>"
  Bus Selector7/3 -> Integrator3/1  "<rl>"

== system Modified/Vehicle/Vehicle/Wheels, Tyres & Suspsension/Springs, Dampers & Linkage/Sum ==
  F_s4 : Inport
  F_d4 : Inport  Port=2
  Bus Creator4 : BusCreator
  Bus Selector7 : BusSelector  OutputSignals=fl,fr,rl,rr
  Bus Selector8 : BusSelector  OutputSignals=fl,fr,rl,rr
  Sum{1..4} (4 alike) : Sum
  F_sd4 : Outport
  wires:
  Sum3/1 -> Bus Creator4/3  "rl"
  Sum4/1 -> Bus Creator4/4  "rr"
  Sum1/1 -> Bus Creator4/1  "fl"
  Sum2/1 -> Bus Creator4/2  "fr"
  Bus Selector8/1 -> Sum1/2  "<fl>"
  F_d4/1 -> Bus Selector8/1
  F_s4/1 -> Bus Selector7/1
  Bus Selector7/3 -> Sum3/1  "<rl>"
  Bus Selector7/4 -> Sum4/1  "<rr>"
  Bus Selector7/2 -> Sum2/1  "<fr>"
  Bus Selector7/1 -> Sum1/1  "<fl>"
  Bus Creator4/1 -> F_sd4/1  "F_sd4"
  Bus Selector8/4 -> Sum4/2  "<rr>"
  Bus Selector8/3 -> Sum3/2  "<rl>"
  Bus Selector8/2 -> Sum2/2  "<fr>"

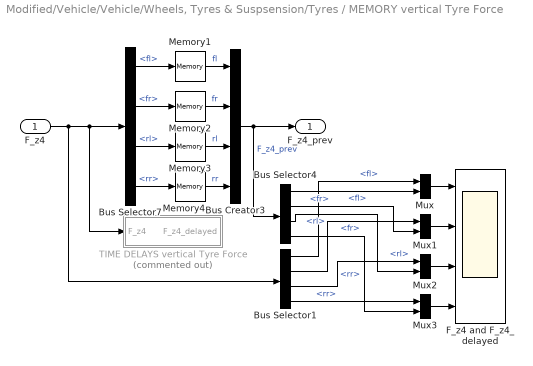
== system Modified/Vehicle/Vehicle/Wheels, Tyres & Suspsension/Tyres / MEMORY vertical Tyre Force ==
  F_z4 : Inport
  Bus Creator3 : BusCreator
  Bus Selector1 : BusSelector  OutputSignals=fl,fr,rl,rr
  Bus Selector4 : BusSelector  OutputSignals=fl,fr,rl,rr
  Bus Selector7 : BusSelector  OutputSignals=fl,fr,rl,rr
  F_z4 and F_z4_delayed : Scope  NumInputPorts=4
      settings: YMin=2000~1000~1000~1000  YMax=9000~8000~6000~5500  SaveName=ScopeData16
  Memory{1..4} (4 alike) : Memory
  Mux{,1..3} (4 alike) : Mux  Inputs=2
  TIME DELAYS vertical Tyre Force : Subsystem  Commented=on
      settings: MinAlgLoopOccurrences=on
  F_z4_prev : Outport
  wires:
  Memory1/1 -> Bus Creator3/1  "fl"
  Memory3/1 -> Bus Creator3/3  "rl"
  Memory4/1 -> Bus Creator3/4  "rr"
  Memory2/1 -> Bus Creator3/2  "fr"
  F_z4/1 -> Bus Selector1/1, TIME DELAYS vertical Tyre Force/1(F_z4), Bus Selector7/1
  Bus Selector7/1 -> Memory1/1  "<fl>"
  Bus Creator3/1 -> Bus Selector4/1, F_z4_prev/1  "F_z4_prev"
  Bus Selector7/2 -> Memory2/1  "<fr>"
  Bus Selector7/4 -> Memory4/1  "<rr>"
  Bus Selector7/3 -> Memory3/1  "<rl>"
  Bus Selector4/1 -> Mux/2  "<fl>"
  Mux/1 -> F_z4 and F_z4_delayed/1
  Bus Selector1/1 -> Mux/1  "<fl>"
  Mux1/1 -> F_z4 and F_z4_delayed/2
  Mux2/1 -> F_z4 and F_z4_delayed/3
  Mux3/1 -> F_z4 and F_z4_delayed/4
  Bus Selector1/2 -> Mux1/1  "<fr>"
  Bus Selector1/3 -> Mux2/1  "<rl>"
  Bus Selector1/4 -> Mux3/1  "<rr>"
  Bus Selector4/3 -> Mux2/2  "<rl>"
  Bus Selector4/4 -> Mux3/2  "<rr>"
  Bus Selector4/2 -> Mux1/2  "<fr>"

== system Modified/Vehicle/Vehicle/Wheels, Tyres & Suspsension/Tyres /INTEGRATOR Tyre Force in ground plane ==
  derF_xyw4 : Inport
  Bus Creator3 : BusCreator
  Bus Selector7 : BusSelector  OutputSignals=fl,fr,rl,rr
  Integrator{1..4} (4 alike) : Integrator
  F_xyw4 : Outport
  wires:
  Integrator1/1 -> Bus Creator3/1  "fl"
  Integrator3/1 -> Bus Creator3/3  "rl"
  Integrator4/1 -> Bus Creator3/4  "rr"
  Integrator2/1 -> Bus Creator3/2  "fr"
  derF_xyw4/1 -> Bus Selector7/1
  Bus Selector7/1 -> Integrator1/1  "<fl>"
  Bus Creator3/1 -> F_xyw4/1  "F_xvw4"
  Bus Selector7/2 -> Integrator2/1  "<fr>"
  Bus Selector7/4 -> Integrator4/1  "<rr>"
  Bus Selector7/3 -> Integrator3/1  "<rl>"

== system Modified/Vehicle/Vehicle/Wheels, Tyres & Suspsension/Wheels /INTEGRATOR ==
  derw_w4 : Inport
  Bus Creator1 : BusCreator
  Bus Selector1 : BusSelector  OutputSignals=fl,fr,rl,rr
  Integ Whl{1..4} (4 alike) : Integrator  InitialCondition=Par.Init.v_x/Par.Veh.Rw
  w_w4 : Outport
  wires:
  Integ Whl1/1 -> Bus Creator1/1  "fl"
  Bus Creator1/1 -> w_w4/1  "w_w4"
  Integ Whl4/1 -> Bus Creator1/4  "rr"
  Integ Whl3/1 -> Bus Creator1/3  "rl"
  Integ Whl2/1 -> Bus Creator1/2  "fr"
  Bus Selector1/4 -> Integ Whl4/1  "<rr>"
  Bus Selector1/2 -> Integ Whl2/1  "<fr>"
  Bus Selector1/1 -> Integ Whl1/1  "<fl>"
  Bus Selector1/3 -> Integ Whl3/1  "<rl>"
  derw_w4/1 -> Bus Selector1/1

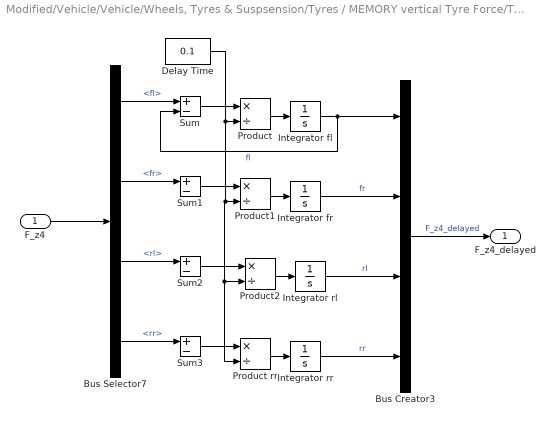
== system Modified/Vehicle/Vehicle/Wheels, Tyres & Suspsension/Tyres / MEMORY vertical Tyre Force/TIME DELAYS vertical Tyre Force ==
  F_z4 : Inport
  Bus Creator3 : BusCreator
  Bus Selector7 : BusSelector  OutputSignals=fl,fr,rl,rr
  Delay Time : Constant  Value=0.1
  Integrator fl : Integrator
  Integrator fr : Integrator
  Integrator rl : Integrator
  Integrator rr : Integrator
  Product : Product  Inputs=*/
  Product rr : Product  Inputs=*/
  Product1 : Product  Inputs=*/
  Product2 : Product  Inputs=*/
  Sum{,1..3} (4 alike) : Sum  Inputs=+-
  F_z4_delayed : Outport
  wires:
  Integrator fl/1 -> Bus Creator3/1, Sum/2  "fl"
  Integrator rl/1 -> Bus Creator3/3  "rl"
  Integrator rr/1 -> Bus Creator3/4  "rr"
  Integrator fr/1 -> Bus Creator3/2  "fr"
  F_z4/1 -> Bus Selector7/1
  Bus Selector7/1 -> Sum/1  "<fl>"
  Bus Creator3/1 -> F_z4_delayed/1  "F_z4_delayed"
  Bus Selector7/2 -> Sum1/1  "<fr>"
  Bus Selector7/4 -> Sum3/1  "<rr>"
  Bus Selector7/3 -> Sum2/1  "<rl>"
  Sum/1 -> Product/1
  Product/1 -> Integrator fl/1
  Delay Time/1 -> Product2/2, Product rr/2, Product1/2, Product/2
  Sum1/1 -> Product1/1
  Product1/1 -> Integrator fr/1
  Sum2/1 -> Product2/1
  Product2/1 -> Integrator rl/1
  Sum3/1 -> Product rr/1
  Product rr/1 -> Integrator rr/1

== matlab function Modified/Vehicle/Vehicle/Wheels, Tyres & Suspsension/Tyres /Tyre Slip ==
  data: w_4 input Bus: whl_vec4; v_xw4 input Bus: whl_vec4; v_yw4 input Bus: whl_vec4; s_x4 output Bus: whl_vec4; s_y4 output Bus: whl_vec4; Par parameter; s_xy4 output Bus: whl_vec4
function [s_x4, s_y4, s_xy4] = TyreModel(w_4, v_xw4, v_yw4, Par)
%#codegen

Rw=Par.Veh.Rw;

s_x4.fl=(Rw*w_4.fl-v_xw4.fl)/(abs(Rw*w_4.fl+v_xw4.fl)/2);
s_x4.fr=(Rw*w_4.fr-v_xw4.fr)/(abs(Rw*w_4.fr+v_xw4.fr)/2);
s_x4.rl=(Rw*w_4.rl-v_xw4.rl)/(abs(Rw*w_4.rl+v_xw4.rl)/2);
s_x4.rr=(Rw*w_4.rr-v_xw4.rr)/(abs(Rw*w_4.rr+v_xw4.rr)/2);

s_y4.fl=v_yw4.fl/(abs(Rw*w_4.fl+v_xw4.fl)/2);
s_y4.fr=v_yw4.fr/(abs(Rw*w_4.fr+v_xw4.fr)/2);
s_y4.rl=v_yw4.rl/(abs(Rw*w_4.rl+v_xw4.rl)/2);
s_y4.rr=v_yw4.rr/(abs(Rw*w_4.rr+v_xw4.rr)/2);

s_xy4.fl=sqrt(s_x4.fl^2+s_y4.fl^2);
s_xy4.fr=sqrt(s_x4.fr^2+s_y4.fr^2);
s_xy4.rl=sqrt(s_x4.rl^2+s_y4.rl^2);
s_xy4.rr=sqrt(s_x4.rr^2+s_y4.rr^2);

== matlab function Modified/Vehicle/Vehicle/Wheels, Tyres & Suspsension/Tyres /Tyre-Slip Force ==
  data: s_xy4 input Bus: whl_vec4; F_xywSS4 output Bus: whl_vec4; F_z4 input Bus: whl_vec4; Par parameter
function F_xywSS4  = TyreModel(s_xy4, F_z4, Par)
%#codegen

C0=Par.Veh.C0; 
mu=Par.Env.mu;
Rw=Par.Veh.Rw;

F_xywSS4.fl = min(C0*s_xy4.fl, mu) * max(F_z4.fl, 0);
F_xywSS4.fr = min(C0*s_xy4.fr, mu) * max(F_z4.fr, 0);
F_xywSS4.rl = min(C0*s_xy4.rl, mu) * max(F_z4.rl, 0);
F_xywSS4.rr = min(C0*s_xy4.rr, mu) * max(F_z4.rr, 0);


% if s_xy4.fl>Par.Env.mu/Par.Veh.C0
%     F_xywSS4.fl=min(C0*s_xy4.fl,mu)*max(F_z4.fl,0);
% else
%     F_xw4.fl=+max(F_z4.fl,0)*Par.Veh.C0*s_x4.fl;
%     F_yw4.fl=-max(F_z4.fl,0)*Par.Veh.C0*s_y4.fl;
% end

== matlab function Modified/Vehicle/Vehicle/Wheels, Tyres & Suspsension/Springs, Dampers & Linkage/Suspension Equilibrium ==
  data: T_s4 input Bus: whl_vec4; F_sd4 input Bus: whl_vec4; F_z4 output Bus: whl_vec4; F_xv4 input Bus: whl_vec4; F_yv4 input Bus: whl_vec4; delta_w4 input Bus: whl_vec4; Par parameter
function F_z4   = SuspEquil(T_s4, F_sd4, F_xv4,F_yv4,delta_w4, Par)
%#codegen

F_z4.fl = F_sd4.fl +(+T_s4.fl*(cos(delta_w4.fl)*Par.Veh.r_lever.fl(2) -Par.Veh.r_lever.fl(1)*sin(delta_w4.fl))...
    -F_xv4.fl*(Par.Veh.r_lever.fl(2)*Par.Veh.r_pivot.fl(3)+Par.Veh.r_lever.fl(3)*Par.Veh.r_pivot.fl(2)) ...
    +F_yv4.fl*(Par.Veh.r_lever.fl(1)*Par.Veh.r_pivot.fl(3)-Par.Veh.r_lever.fl(3)*Par.Veh.r_pivot.fl(1))) ...
    /(Par.Veh.r_lever.fl(1)*Par.Veh.r_pivot.fl(2)-Par.Veh.r_lever.fl(2)*Par.Veh.r_pivot.fl(1));
F_z4.fr = F_sd4.fr +(+T_s4.fr*(cos(delta_w4.fr)*Par.Veh.r_lever.fr(2) -Par.Veh.r_lever.fr(1)*sin(delta_w4.fr))...
    -F_xv4.fr*(Par.Veh.r_lever.fr(2)*Par.Veh.r_pivot.fr(3)+Par.Veh.r_lever.fr(3)*Par.Veh.r_pivot.fr(2)) ...
    +F_yv4.fr*(Par.Veh.r_lever.fr(1)*Par.Veh.r_pivot.fr(3)-Par.Veh.r_lever.fr(3)*Par.Veh.r_pivot.fr(1))) ...
    /(Par.Veh.r_lever.fr(1)*Par.Veh.r_pivot.fr(2)-Par.Veh.r_lever.fr(2)*Par.Veh.r_pivot.fr(1));
F_z4.rl = F_sd4.rl +(+T_s4.rl*(cos(delta_w4.rl)*Par.Veh.r_lever.rl(2) -Par.Veh.r_lever.rl(1)*sin(delta_w4.rl))...
    -F_xv4.rl*(Par.Veh.r_lever.rl(2)*Par.Veh.r_pivot.rl(3)+Par.Veh.r_lever.rl(3)*Par.Veh.r_pivot.rl(2)) ...
    +F_yv4.rl*(Par.Veh.r_lever.rl(1)*Par.Veh.r_pivot.rl(3)-Par.Veh.r_lever.rl(3)*Par.Veh.r_pivot.rl(1))) ...
    /(Par.Veh.r_lever.rl(1)*Par.Veh.r_pivot.rl(2)-Par.Veh.r_lever.rl(2)*Par.Veh.r_pivot.rl(1));
F_z4.rr = F_sd4.rr +(+T_s4.rr*(cos(delta_w4.rr)*Par.Veh.r_lever.rr(2) -Par.Veh.r_lever.rr(1)*sin(delta_w4.rr))...
    -F_xv4.rr*(Par.Veh.r_lever.rr(2)*Par.Veh.r_pivot.rr(3)+Par.Veh.r_lever.rr(3)*Par.Veh.r_pivot.rr(2)) ...
    +F_yv4.rr*(Par.Veh.r_lever.rr(1)*Par.Veh.r_pivot.rr(3)-Par.Veh.r_lever.rr(3)*Par.Veh.r_pivot.rr(1))) ...
    /(Par.Veh.r_lever.rr(1)*Par.Veh.r_pivot.rr(2)-Par.Veh.r_lever.rr(2)*Par.Veh.r_pivot.rr(1));

% h1f=Par.Veh.hf;
% h2f=h1f;
% h3f=Par.Veh.hf;
% h4f=h3f;
% 
% f1=Par.Veh.ff;
% f2=-f1;
% f3=Par.Veh.fr;
% f4=-f3;
% 
% F_z4.fl=(0*F_xv4.fl +h1f*F_yv4.fl +0*T_s4.fl +(-f1)*F_sd4.fl)/(-f1);
% F_z4.fr=(0*F_xv4.fr +h2f*F_yv4.fr +0*T_s4.fr +(-f2)*F_sd4.fr)/(-f2);
% F_z4.rl=(0*F_xv4.rl +h3f*F_yv4.rl +0*T_s4.rl +(-f3)*F_sd4.rl)/(-f3);
% F_z4.rr=(0*F_xv4.rr +h4f*F_yv4.rr +0*T_s4.rr +(-f4)*F_sd4.rr)/(-f4);

== matlab function Modified/Vehicle/Vehicle/Wheels, Tyres & Suspsension/Tyres /Tyre Relaxation ==
  data: w_4 input Bus: whl_vec4; F_xywSS4 input; derF_xyw4 output Bus: whl_vec4; F_xyw4 input Bus: whl_vec4; Par parameter
function derF_xyw4   = TyreModel(w_4, F_xywSS4, F_xyw4, Par)
%#codegen

derF_xyw4.fl=(F_xywSS4.fl-F_xyw4.fl)*abs(Par.Veh.Rw*w_4.fl)/Par.Veh.RelaxLength;
derF_xyw4.fr=(F_xywSS4.fr-F_xyw4.fr)*abs(Par.Veh.Rw*w_4.fr)/Par.Veh.RelaxLength;
derF_xyw4.rl=(F_xywSS4.rl-F_xyw4.rl)*abs(Par.Veh.Rw*w_4.rl)/Par.Veh.RelaxLength;
derF_xyw4.rr=(F_xywSS4.rr-F_xyw4.rr)*abs(Par.Veh.Rw*w_4.rr)/Par.Veh.RelaxLength;

== matlab function Modified/Vehicle/Vehicle/Vehicle Motion/Whole Vehicle IRP/Vehicle Velocity in-road-plane ==
  data: F_xv4 input Bus: whl_vec4; F_yv4 input Bus: whl_vec4; v_irp3 input Bus: irp_vec3; Par parameter; derv_irp3 output Bus: irp_vec3
function derv_irp3  = Body_irp(F_xv4,F_yv4, v_irp3, Par)
%old: function derv_irp3  = Body_irp(F_1xv,F_2xv,F_3xv,F_4xv, F_1yv,F_2yv,F_3yv,F_4yv, v_irp3, Par)
%#codegen

v_x=v_irp3.x;
v_y=v_irp3.y;
w_z=v_irp3.rotz;

lf=Par.Veh.lf;
lr=Par.Veh.lr;

w1=Par.Veh.TrackWidth/2;
w2=-w1;
w3=w1;
w4=-w3;

T_irpv=[[ 1   1   1   1 ] [0  0  0  0 ]; ...
    [ 0   0   0   0 ] [1  1  1  1 ]; ...
    [-w1 -w2 -w3 -w4] [lf lf lr lr]];

F_xv4_temp=[F_xv4.fl;F_xv4.fr;F_xv4.rl;F_xv4.rr];
F_yv4_temp=[F_yv4.fl;F_yv4.fr;F_yv4.rl;F_yv4.rr];

F_air=Par.Veh.HalfRohACd*abs(v_x)*v_x;
beta=atan2(v_y,v_x);

derv_irp3_temp=diag([1/Par.Veh.m 1/Par.Veh.m 1/Par.Veh.Jz])*(T_irpv*[F_xv4_temp;F_yv4_temp]-[sin(beta);sin(beta);0]*F_air)-[-v_y*w_z; +v_x*w_z; 0];

derv_irp3 = struct('x',derv_irp3_temp(1),'y',derv_irp3_temp(2),'rotz',derv_irp3_temp(3));

== matlab function Modified/Vehicle/Vehicle/Vehicle Motion/Whole Vehicle IRP/Vehicle Position in-road-plane ==
  data: v_irp3 input Bus: irp_vec3; p_z input; derpos_irp3 output Bus: irp_vec3
function derpos_irp3  = BodyPath_irp(v_irp3, p_z)
%#codegen

derpos_irp3.x   = cos(p_z)*v_irp3.x -sin(p_z)*v_irp3.y;
derpos_irp3.y   = sin(p_z)*v_irp3.x +cos(p_z)*v_irp3.y;
derpos_irp3.rotz= v_irp3.rotz;

== matlab function Modified/Vehicle/Vehicle/Wheels, Tyres & Suspsension/Springs, Dampers & Linkage/Dampers ==
  data: v_z4 input Bus: whl_vec4; F_d4 output Bus: whl_vec4; Par parameter
function F_d4   =  Dampers(v_z4,Par)
%old: function [F_1d,F_2d,F_3d,F_4d]  =  Dampers(v_1z,v_2z,v_3z,v_4z,Par)
%#codegen

d1=Par.Veh.dw;
d2=Par.Veh.dw;
d3=Par.Veh.dw;
d4=Par.Veh.dw;

F_d4.fl=-d1*v_z4.fl;
F_d4.fr=-d2*v_z4.fr;
F_d4.rl=-d3*v_z4.rl;
F_d4.rr=-d4*v_z4.rr;

== matlab function Modified/Vehicle/Vehicle/Wheels, Tyres & Suspsension/Springs, Dampers & Linkage/Springs ==
  data: v_z4 input Bus: whl_vec4; derF_s4 output Bus: whl_vec4; Par parameter
function derF_s4   = Springs(v_z4,Par)
%old: function [derF_1s,derF_2s,derF_3s,derF_4s]  = Springs(v_1z,v_2z,v_3z,v_4z,Par)
%#codegen

derF_s4.fl=[Par.Veh.cw, Par.Veh.carb_f]*[-v_z4.fl; -v_z4.fr];
derF_s4.fr=[Par.Veh.cw, Par.Veh.carb_f]*[-v_z4.fr; -v_z4.fl];
derF_s4.rl=[Par.Veh.cw, Par.Veh.carb_r]*[-v_z4.rl; -v_z4.rr];
derF_s4.rr=[Par.Veh.cw, Par.Veh.carb_r]*[-v_z4.rr; -v_z4.rl];

== matlab function Modified/Vehicle/Vehicle/Vehicle Motion/Sprung Body OORP/Body OORP ==
  data: F_xv4 input Bus: whl_vec4; derv_oorp3 output Bus: oorp_vec3; F_yv4 input Bus: whl_vec4; F_z4 input Bus: whl_vec4; Par parameter
function derv_oorp3   = fcn(F_xv4,F_yv4, F_z4, Par)
%old: function derv_oorp3   = fcn(F_1xv,F_2xv,F_3xv,F_4xv, F_1yv,F_2yv,F_3yv,F_4yv, F_1z,F_2z,F_3z,F_4z, Par)
%#codegen

w1=Par.Veh.TrackWidth/2; %"half wheel base" #Can notation w1 conflict with wheel rotational speed?
w2=-w1;
w3=w1;
w4=w2;

lf=Par.Veh.lf;
lr=Par.Veh.lr;

h=Par.Veh.h; 

T_oorpv=[[ 1   1   1   1 ];...
         [ w1  w2  w3  w4];...
         [-lf -lf -lr -lr]];

F_xv4_temp=[F_xv4.fl;F_xv4.fr;F_xv4.rl;F_xv4.rr];
F_yv4_temp=[F_yv4.fl;F_yv4.fr;F_yv4.rl;F_yv4.rr];
F_z4_temp =[F_z4.fl; F_z4.fr; F_z4.rl; F_z4.rr];

     
F_oorp3=...
[[0 0 0 0; 0 0 0 0; -h -h -h -h]*F_xv4_temp+...
 [0 0 0 0; h h h h;  0  0  0  0]*F_yv4_temp+...
 T_oorpv*F_z4_temp]+[-Par.Veh.m*Par.Env.g;0;0];

derv_oorp3.z=F_oorp3(1)/Par.Veh.m_sprung;
derv_oorp3.rotx=F_oorp3(2)/Par.Veh.Jx_sprung;
derv_oorp3.roty=F_oorp3(3)/Par.Veh.Jy_sprung;

== matlab function Modified/Vehicle/Vehicle/Vehicle Motion/Compatibility IRP/Compatibility ==
  data: v_xv4 output Bus: whl_vec4; v_yv4 output Bus: whl_vec4; v_irp3 input Bus: irp_vec3; Par parameter
function [v_xv4,v_yv4] = fcn(v_irp3,Par)
%old: function [v_1xv,v_2xv,v_3xv,v_4xv, v_1yv,v_2yv,v_3yv,v_4yv] = fcn(v_x,v_y,w_z,Par)
%#codegen

lf=Par.Veh.lf;
lr=Par.Veh.lr;

w1=Par.Veh.TrackWidth/2;
w2=-w1;
w3=w1;
w4=-w3;

T_irpv=[[ 1   1   1   1 ] [0  0  0  0 ]; ...
        [ 0   0   0   0 ] [1  1  1  1 ]; ...
        [-w1 -w2 -w3 -w4] [lf lf lr lr]];

v_irp3_temp=[v_irp3.x; v_irp3.y; v_irp3.rotz];
 
v_xyv8=T_irpv'*v_irp3_temp;

v_xv4=struct('fl',v_xyv8(1),'fr',v_xyv8(2),'rl',v_xyv8(3),'rr',v_xyv8(4));
v_yv4=struct('fl',v_xyv8(5),'fr',v_xyv8(6),'rl',v_xyv8(7),'rr',v_xyv8(8));

== matlab function Modified/Vehicle/Vehicle/Vehicle Motion/Compatibility OORP/Compatibility Eq [1.11] ==
  data: v_oorp3 input Bus: oorp_vec3; v_z4 output Bus: whl_vec4; Par parameter
function v_z4  = fcn(v_oorp3,Par)
%old: function [v_1z,v_2z,v_3z,v_4z] = fcn(v_z,w_x,w_y,Par)
%#codegen

w1=Par.Veh.TrackWidth/2;
w2=-w1;
w3=w1;
w4=w2;

lf=Par.Veh.lf;
lr=Par.Veh.lr;

v_oorp3_temp=[v_oorp3.z; v_oorp3.rotx; v_oorp3.roty];

v_oorp4=[[1;1;1;1] [w1;w2;w3;w4] [-lf;-lf;-lr;-lr]]*v_oorp3_temp;

v_z4=struct('fl',v_oorp4(1),'fr',v_oorp4(2),'rl',v_oorp4(3),'rr',v_oorp4(4));

== matlab function Modified/Vehicle/Vehicle/Wheels, Tyres & Suspsension/Tyres /Tyre Force Direction ==
  data: s_x4 input Bus: whl_vec4; s_y4 input Bus: whl_vec4; s_xy4 input; F_xyw4 input Bus: whl_vec4; F_z4_prev input Bus: whl_vec4; F_xw4 output Bus: whl_vec4; F_yw4 output Bus: whl_vec4; Par parameter
function [F_xw4,F_yw4]  = TyreModel(s_x4, s_y4, s_xy4, F_xyw4, F_z4_prev, Par)
%#codegen

F_z4_temp=[F_z4_prev.fl; F_z4_prev.fr; F_z4_prev.rl; F_z4_prev.rr];
%F_z4_temp=[Par.Veh.F_z4_static(1); Par.Veh.F_z4_static(2); Par.Veh.F_z4_static(3); Par.Veh.F_z4_static(4)];

if s_xy4.fl>Par.Env.mu/Par.Veh.C0
    F_xw4.fl=F_xyw4.fl*(+s_x4.fl/s_xy4.fl);
    F_yw4.fl=F_xyw4.fl*(-s_y4.fl/s_xy4.fl);
else
    F_xw4.fl=+F_z4_temp(1)*Par.Veh.C0*s_x4.fl; %I tried Par.Veh.F_z4_static(1) instead of F_z4.fl but too dis-continous
    F_yw4.fl=-F_z4_temp(1)*Par.Veh.C0*s_y4.fl;
end

if s_xy4.fr>Par.Env.mu/Par.Veh.C0
    F_xw4.fr=F_xyw4.fr*(+s_x4.fr/s_xy4.fr);
    F_yw4.fr=F_xyw4.fr*(-s_y4.fr/s_xy4.fr);
else
    F_xw4.fr=+F_z4_temp(2)*Par.Veh.C0*s_x4.fr;
    F_yw4.fr=-F_z4_temp(2)*Par.Veh.C0*s_y4.fr;
end

if s_xy4.rl>Par.Env.mu/Par.Veh.C0
    F_xw4.rl=F_xyw4.rl*(+s_x4.rl/s_xy4.rl);
    F_yw4.rl=F_xyw4.rl*(-s_y4.rl/s_xy4.rl);
else
    F_xw4.rl=+F_z4_temp(3)*Par.Veh.C0*s_x4.rl;
    F_yw4.rl=-F_z4_temp(3)*Par.Veh.C0*s_y4.rl;
end

if s_xy4.rr>Par.Env.mu/Par.Veh.C0
    F_xw4.rr=F_xyw4.rr*(+s_x4.rr/s_xy4.rr);
    F_yw4.rr=F_xyw4.rr*(-s_y4.rr/s_xy4.rr);
else
    F_xw4.rr=+F_z4_temp(4)*Par.Veh.C0*s_x4.rr;
    F_yw4.rr=-F_z4_temp(4)*Par.Veh.C0*s_y4.rr;
end

% if s_xy4.fl>Par.Env.mu/Par.Veh.C0
%     F_xw4.fl=F_xyw4.fl*(+s_x4.fl/s_xy4.fl);
%     F_yw4.fl=F_xyw4.fl*(-s_y4.fl/s_xy4.fl);
% else
%     F_xw4.fl=+max(F_z4.fl,0)*Par.Veh.C0*s_x4.fl;
%     F_yw4.fl=-max(F_z4.fl,0)*Par.Veh.C0*s_y4.fl;
% end
% 
% if s_xy4.fr>Par.Env.mu/Par.Veh.C0
%     F_xw4.fr=F_xyw4.fr*(+s_x4.fr/s_xy4.fr);
%     F_yw4.fr=F_xyw4.fr*(-s_y4.fr/s_xy4.fr);
% else
%     F_xw4.fr=+max(F_z4.fr,0)*Par.Veh.C0*s_x4.fr;
%     F_yw4.fr=-max(F_z4.fr,0)*Par.Veh.C0*s_y4.fr;
% end
% 
% if s_xy4.rl>Par.Env.mu/Par.Veh.C0
%     F_xw4.rl=F_xyw4.rl*(+s_x4.rl/s_xy4.rl);
%     F_yw4.rl=F_xyw4.rl*(-s_y4.rl/s_xy4.rl);
% else
%     F_xw4.rl=+max(F_z4.rl,0)*Par.Veh.C0*s_x4.rl;
%     F_yw4.rl=-max(F_z4.rl,0)*Par.Veh.C0*s_y4.rl;
% end
% 
% if s_xy4.rr>Par.Env.mu/Par.Veh.C0
%     F_xw4.rr=F_xyw4.rr*(+s_x4.rr/s_xy4.rr);
%     F_yw4.rr=F_xyw4.rr*(-s_y4.rr/s_xy4.rr);
% else
%     F_xw4.rr=+max(F_z4.rr,0)*Par.Veh.C0*s_x4.rr;
%     F_yw4.rr=-max(F_z4.rr,0)*Par.Veh.C0*s_y4.rr;
% end


% F_xw4.fl=-F_xyw4.fl*cos(atan2(s_y4.fl,-s_x4.fl));
% F_xw4.fr=-F_xyw4.fr*cos(atan2(s_y4.fr,-s_x4.fr));
% F_xw4.rl=-F_xyw4.rl*cos(atan2(s_y4.rl,-s_x4.rl));
% F_xw4.rr=-F_xyw4.rr*cos(atan2(s_y4.rr,-s_x4.rr));
% 
% F_yw4.fl=-F_xyw4.fl*sin(atan2(s_y4.fl,-s_x4.fl));
% F_yw4.fr=-F_xyw4.fr*sin(atan2(s_y4.fr,-s_x4.fr));
% F_yw4.rl=-F_xyw4.rl*sin(atan2(s_y4.rl,-s_x4.rl));
% F_yw4.rr=-F_xyw4.rr*sin(atan2(s_y4.rr,-s_x4.rr));
